simulink subsystem "IMUSensor"  (R2025a)
settings: Solver=VariableStepAuto  StartTime=0.0  StopTime=10.0  RelTol=1e-3
libraries: autolibsharedcommon x2, vehdynlibsens x1
settings Model: ModifiedByFormat=The MathWorks, Inc.  Creator=The MathWorks, Inc.  LastModifiedBy=The MathWorks, Inc.
settings RTWCC: GPUComputeCapability=3.5

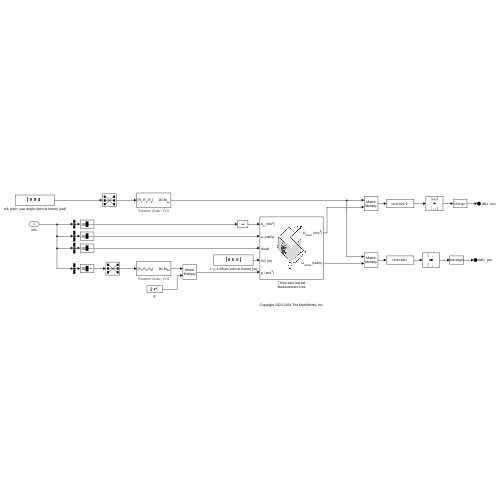
[thumbnail: Simulink's stored preview of the top-level diagram]
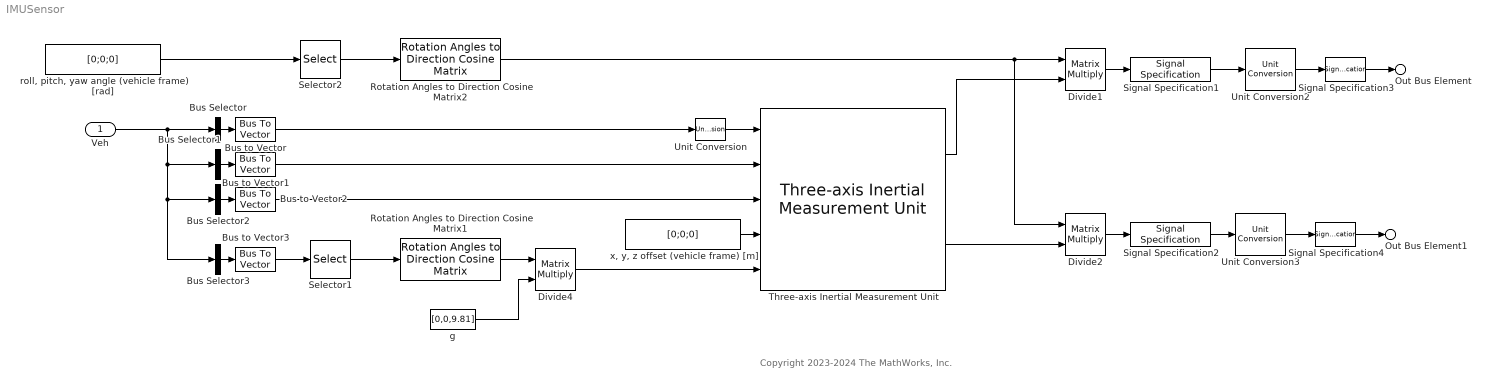
== system IMUSensor ==
  note: Copyright 2023-2024 The MathWorks, Inc.
  Veh : Inport
  Bus Selector : BusSelector  OutputSignals=BdyFrm.Cg.Acc.ax,BdyFrm.Cg.Acc.ay,BdyFrm.Cg.Acc.az  OutputAsBus=on
  Bus Selector1 : BusSelector  OutputSignals=BdyFrm.Cg.AngVel.p,BdyFrm.Cg.AngVel.q,BdyFrm.Cg.AngVel.r  OutputAsBus=on
  Bus Selector2 : BusSelector  OutputSignals=BdyFrm.Cg.AngAcc.pdot,BdyFrm.Cg.AngAcc.qdot,BdyFrm.Cg.AngAcc.rdot  OutputAsBus=on
  Bus Selector3 : BusSelector  OutputSignals=InertFrm.Cg.Ang.phi,InertFrm.Cg.Ang.theta,InertFrm.Cg.Ang.psi  OutputAsBus=on
  Bus to Vector{,1..3} (4 alike) : BusToVector
  Divide1 : Product  Inputs=**  Multiplication=Matrix(*)
  Divide2 : Product  Inputs=**  Multiplication=Matrix(*)
  Divide4 : Product  Inputs=**  Multiplication=Matrix(*)
  Rotation Angles to Direction Cosine Matrix1 : autolibsharedcommon/Rotation Angles to Direction Cosine Matrix  rotationOrder=ZYX  aMode=aMode
      settings: AttributesFormatString=Rotation Order: %<rotationOrder>
  Rotation Angles to Direction Cosine Matrix2 : autolibsharedcommon/Rotation Angles to Direction Cosine Matrix  rotationOrder=ZYX  aMode=aMode
      settings: AttributesFormatString=Rotation Order: %<rotationOrder>
  Selector1 : Selector  InputPortWidth=3  IndexOptions=Index vector (dialog)  Indices=[3 2 1]  OutputSizes=1
  Selector2 : Selector  InputPortWidth=3  IndexOptions=Index vector (dialog)  Indices=[3 2 1]  OutputSizes=1
  Signal Specification1 : SignalSpecification  Unit=m/s^2
  Signal Specification2 : SignalSpecification  Unit=rad/s
  Signal Specification3 : SignalSpecification  Unit=gn
  Signal Specification4 : SignalSpecification  Unit=deg/s
  Three-axis Inertial Measurement Unit : vehdynlibsens/Three-axis Inertial Measurement Unit  units=Metric (MKS)  imu=[0 0 0]  i_Ts=0  dtype_a=off  w_a=190  z_a=0.707  a_sf_cc=[1 0 0; 0 1 0; 0 0 1]  a_bias=[0 0 0]  a_sat="[-inf  -inf  -inf  inf inf inf]"  dtype_g=off  w_g=190  z_g=0.707  g_sf_cc=[1 0 0; 0 1 0; 0 0 1]  g_bias=[0 0 0]  g_sens=[0 0 0]  g_sat="[-inf  -inf  -inf  inf inf inf]"  i_rand=on  i_seeds=[23093 23094 23095 23096 23097 23098]  i_pow=[0.001 0.001 0.001 0.0001 0.0001 0.0001]  aMode=2
  Unit Conversion : UnitConversion
  Unit Conversion2 : UnitConversion
  Unit Conversion3 : UnitConversion
  g : Constant  Value=[0,0,9.81]
  "roll, pitch, yaw angle (vehicle frame) [rad]" : Constant  Value=[0;0;0]
  "x, y, z offset (vehicle frame) [m]" : Constant  Value=[0;0;0]
  Out Bus Element : Outport  PortName=IMU  Element=Acc
  Out Bus Element1 : Outport  PortName=IMU  Element=pqr
  wires:
  Unit Conversion/1 -> Three-axis Inertial Measurement Unit/1
  "x, y, z offset (vehicle frame) [m]"/1 -> Three-axis Inertial Measurement Unit/4
  Bus Selector2/1 -> Bus to Vector2/1
  Signal Specification3/1 -> Out Bus Element/1
  Bus to Vector2/1 -> Three-axis Inertial Measurement Unit/3
  Bus Selector/1 -> Bus to Vector/1
  Bus to Vector1/1 -> Three-axis Inertial Measurement Unit/2
  Bus Selector1/1 -> Bus to Vector1/1
  Bus to Vector/1 -> Unit Conversion/1
  g/1 -> Divide4/2
  Veh/1 -> Bus Selector/1, Bus Selector1/1, Bus Selector2/1, Bus Selector3/1
  Bus Selector3/1 -> Bus to Vector3/1
  Rotation Angles to Direction Cosine Matrix1/1 -> Divide4/1
  Selector1/1 -> Rotation Angles to Direction Cosine Matrix1/1
  Bus to Vector3/1 -> Selector1/1
  Three-axis Inertial Measurement Unit/2 -> Divide2/2
  Unit Conversion3/1 -> Signal Specification4/1
  Unit Conversion2/1 -> Signal Specification3/1
  Signal Specification4/1 -> Out Bus Element1/1
  Divide2/1 -> Signal Specification2/1
  Divide1/1 -> Signal Specification1/1
  Rotation Angles to Direction Cosine Matrix2/1 -> Divide2/1, Divide1/1
  Signal Specification1/1 -> Unit Conversion2/1
  Signal Specification2/1 -> Unit Conversion3/1
  Three-axis Inertial Measurement Unit/1 -> Divide1/2
  Divide4/1 -> Three-axis Inertial Measurement Unit/5
  Selector2/1 -> Rotation Angles to Direction Cosine Matrix2/1
  "roll, pitch, yaw angle (vehicle frame) [rad]"/1 -> Selector2/1
